simulink model "OMAP_ver_MIL10"  (R2018b)
settings: Solver=FixedStepDiscrete  StartTime=0.0  StopTime=10.0  FixedStep=0.01  RelTol=1e-3
undefined symbols (not defined in the file or in its folder): OMAP_Switch_EMS, OMAP_Switch_EPS, OMAP_Switch_ESC, OMAP_Switch_IC, OMAP_Switch_OTHER, TH_HMIClb_tiDgrdIconWarnHiDurT_C, TH_HMIClb_tiDgrdIconWarnLoDurT_C, TH_HMIClb_tiDgrdVocWarnDurT_C, TH_HMIClb_tiHndOffTxtWarnT_C, TH_HMIClb_tiHndOffVocWarnT_C, TH_HMIClb_tiSWALimFlgDetT_C, TH_HMIClb_tiTxtLimT_C
libraries: simulink x118
(part 6 of 9)

== system OMAP_ver_MIL10/OMAP_Module/ICA_Direct_G59/ICA_Define/TH_HMIClb ==
  note: Level: 3
      | Num: THC.06
      | Rev: 00.00.01
      | Ud: 19-03-28
  Bus Creator1 : BusCreator  Inputs=15
  Constant : Constant  Value=0.01  OutDataTypeStr=single
  Data Type Conversion{,1..7} (8 alike) : DataTypeConversion  OutDataTypeStr=single
  Data Type Conversion{10..13} (4 alike) : DataTypeConversion  OutDataTypeStr=uint16
  ISA_TYPE : Subsystem
      mask Display:
      | port_label('input', 1, 'In');
      | port_label('output', 1, 'Out');
      | color('blue');
      | text(0.5,0.5,'0.789','horizontalAlignment','center');
  ISA_Value : Subsystem
      mask Display:
      | port_label('input', 1, 'In');
      | port_label('output', 1, 'Out');
      | color('blue');
      | text(0.5,0.5,'0.789','horizontalAlignment','center');
  LCScene_tmp : Subsystem
      mask Display:
      | port_label('input', 1, 'In');
      | port_label('output', 1, 'Out');
      | color('blue');
      | text(0.5,0.5,'0.789','horizontalAlignment','center');
  Mode_tmp : Subsystem
      mask Display:
      | port_label('input', 1, 'In');
      | port_label('output', 1, 'Out');
      | color('blue');
      | text(0.5,0.5,'0.789','horizontalAlignment','center');
  TH_HMIClb_tiDgrdIconWarnHiDurT_C : Subsystem
      mask Display:
      | port_label('input', 1, 'In');
      | port_label('output', 1, 'Out');
      | color('blue');
      | text(0.5,0.5,'0.789','horizontalAlignment','center');
  TH_HMIClb_tiDgrdIconWarnLoDurT_C : Subsystem
      mask Display:
      | port_label('input', 1, 'In');
      | port_label('output', 1, 'Out');
      | color('blue');
      | text(0.5,0.5,'0.789','horizontalAlignment','center');
  TH_HMIClb_tiDgrdVocWarnDurT_C : Subsystem
      mask Display:
      | port_label('input', 1, 'In');
      | port_label('output', 1, 'Out');
      | color('blue');
      | text(0.5,0.5,'0.789','horizontalAlignment','center');
  "TH_HMIClb_tiHndOffTxtWarnT_C " : Subsystem
      mask Display:
      | port_label('input', 1, 'In');
      | port_label('output', 1, 'Out');
      | color('blue');
      | text(0.5,0.5,'0.789','horizontalAlignment','center');
  TH_HMIClb_tiHndOffVocWarnT_C : Subsystem
      mask Display:
      | port_label('input', 1, 'In');
      | port_label('output', 1, 'Out');
      | color('blue');
      | text(0.5,0.5,'0.789','horizontalAlignment','center');
  TH_HMIClb_tiSWALimFlgDetT_C : Subsystem
      mask Display:
      | port_label('input', 1, 'In');
      | port_label('output', 1, 'Out');
      | color('blue');
      | text(0.5,0.5,'0.789','horizontalAlignment','center');
  TH_HMIClb_tiTxtLimT_C : Subsystem
      mask Display:
      | port_label('input', 1, 'In');
      | port_label('output', 1, 'Out');
      | color('blue');
      | text(0.5,0.5,'0.789','horizontalAlignment','center');
  Out : Outport
  wires:
  Bus Creator1/1 -> Out/1
  "TH_HMIClb_tiHndOffTxtWarnT_C "/1(Out1) -> Bus Creator1/1  "TH_HMIClb_tiHndOffTxtWarnT_C"
  Data Type Conversion3/1 -> "TH_HMIClb_tiHndOffTxtWarnT_C "/1(In2)
  TH_HMIClb_tiHndOffVocWarnT_C/1(Out1) -> Bus Creator1/2  "TH_HMIClb_tiHndOffVocWarnT_C"
  Data Type Conversion1/1 -> TH_HMIClb_tiHndOffVocWarnT_C/1(In2)
  TH_HMIClb_tiDgrdVocWarnDurT_C/1(Out1) -> Bus Creator1/3  "TH_HMIClb_tiDgrdVocWarnDurT_C"
  Data Type Conversion2/1 -> TH_HMIClb_tiDgrdVocWarnDurT_C/1(In2)
  TH_HMIClb_tiTxtLimT_C/1(Out1) -> Bus Creator1/4  "TH_HMIClb_tiTxtLimT_C"
  Data Type Conversion4/1 -> TH_HMIClb_tiTxtLimT_C/1(In2)
  Data Type Conversion/1 -> Bus Creator1/5  "TH_HMIClb_tiCalcPer_C"
  TH_HMIClb_tiDgrdIconWarnHiDurT_C/1(Out1) -> Bus Creator1/6  "TH_HMIClb_tiDgrdIconWarnHiDurT_C"
  Data Type Conversion5/1 -> TH_HMIClb_tiDgrdIconWarnHiDurT_C/1(In2)
  TH_HMIClb_tiDgrdIconWarnLoDurT_C/1(Out1) -> Bus Creator1/7  "TH_HMIClb_tiDgrdIconWarnLoDurT_C"
  Data Type Conversion6/1 -> TH_HMIClb_tiDgrdIconWarnLoDurT_C/1(In2)
  TH_HMIClb_tiSWALimFlgDetT_C/1(Out1) -> Bus Creator1/8  "TH_HMIClb_tiSWALimFlgDetT_C"
  Data Type Conversion7/1 -> TH_HMIClb_tiSWALimFlgDetT_C/1(In2)
  LCScene_tmp/1(Out1) -> Bus Creator1/11  "LCScene_tmp"
  Data Type Conversion10/1 -> LCScene_tmp/1(In2)  "LCScene_tmp"
  Data Type Conversion12/1 -> ISA_TYPE/1(In2)  "ISA_TYPE"
  ISA_TYPE/1(Out1) -> Bus Creator1/13  "ISA_TYPE"
  ISA_Value/1(Out1) -> Bus Creator1/14  "ISA_Value"
  Data Type Conversion13/1 -> ISA_Value/1(In2)  "ISA_Value"
  Mode_tmp/1(Out1) -> Bus Creator1/15  "Mode_tmp"
  Data Type Conversion11/1 -> Mode_tmp/1(In2)
  Constant/1 -> Data Type Conversion/1

== system OMAP_ver_MIL10/OMAP_Module/ACCS_Direct/ACCS_Define/ACC_State_Synthesis(ACC_SS)/If Action Subsystem2 ==
  In1 : Inport
  Action Port : ActionPort  InitializeStates=reset
  Bus Creator : BusCreator  Inputs=15
  Constant : Constant  Value=2.05  OutDataTypeStr=single
  Constant1 : Constant  Value=6.2  OutDataTypeStr=single
  Constant{3,5,7,9..10} (5 alike) : Constant  Value=0  OutDataTypeStr=uint8
  Constant2 : Constant  Value=6.2  OutDataTypeStr=single
  Constant4 : Constant  Value=-4000  OutDataTypeStr=single
  Constant6 : Constant  Value=-4000  OutDataTypeStr=single
  OMAPve_y_ADAS_ACCRequestEPBNum1 : Constant  Value=0  OutDataTypeStr=uint8
  OMAPve_y_ADAS_ESCDriveOffNum : Constant  Value=0  OutDataTypeStr=uint8
  OMAPve_y_ADAS_ESCHoldReq : Constant  Value=0  OutDataTypeStr=uint8
  Signal Conversion : SignalConversion  OverrideOpt=off
  Subsystem : Subsystem
  Subsystem4 : Subsystem
  Control_Ouput : Outport
  wires:
  Signal Conversion/1 -> Control_Ouput/1
  Constant5/1 -> Bus Creator/12  "Power_steering_power_cut3F2"
  Bus Creator/1 -> Signal Conversion/1
  Subsystem/1(Function_Acc_status) -> Bus Creator/6  "Function_Acc_status"
  In1/1 -> Subsystem/1(In1)
  Constant10/1 -> Bus Creator/11  "MDD_deceleration_type"
  Constant9/1 -> Bus Creator/10  "MDD_Decelerationcontrol_request"
  Subsystem4/1(TYPE_RAPPORT) -> Bus Creator/9  "TYPE_RAPPORT"
  Constant7/1 -> Bus Creator/8  "Powertrain_torquewheel_request"
  Constant6/1 -> Bus Creator/7  "ACCTqReq"
  Constant4/1 -> Bus Creator/5  "PotACCTqReq"
  Constant3/1 -> Bus Creator/4  "StAcvTqWhlPTPotReq"
  Constant2/1 -> Bus Creator/3  "TminUpGear"
  Constant1/1 -> Bus Creator/2  "TminDownGear"
  Constant/1 -> Bus Creator/1  "Deceleration_setpoint_device"
  OMAPve_y_ADAS_ESCDriveOffNum/1 -> Bus Creator/13  "OMAPve_y_ADAS_ESCDriveOff"
  OMAPve_y_ADAS_ESCHoldReq/1 -> Bus Creator/14  "OMAPve_y_ADAS_ESCHoldReq"
  OMAPve_y_ADAS_ACCRequestEPBNum1/1 -> Bus Creator/15  "OMAPve_y_ADAS_ACCRequestEPB"

== system OMAP_ver_MIL10/OMAP_Module/ACCS_Direct/ACCS_Define/ACC_State_Synthesis(ACC_SS)/If Action Subsystem3 ==
  ACT_Control_Signal : Inport
  Action Port : ActionPort  InitializeStates=reset
  Bus Creator : BusCreator  Inputs=15
  Bus Selector1 : BusSelector  OutputSignals=ACCSve_g_ACC_TqReq_convert,ACCSve_d_ACC_TqFlag_convert,ACCSve_g_ACC_DecReq_convert,ACCSve_d_ACC_DecFlag_convert,ACCSve_d_ACC_State_convert,ACCSve_d_ACC_ESCDriveOff_convert,ACCSve_d_ACC_ESCHoldReq_convert,ACCSve_d_ACC_EPBReq_convert
  Constant5 : Constant  Value=0  OutDataTypeStr=uint8
  Data Type Conversion{,1..6} (7 alike) : DataTypeConversion  OutDataTypeStr=uint8
  Gain : Gain  OutDataTypeStr=single
  Signal Conversion : SignalConversion  OverrideOpt=off
  Subsystem : Subsystem
  Subsystem1 : Subsystem
  Subsystem2 : Subsystem
  Subsystem3 : Subsystem
  Subsystem5 : Subsystem
  Subsystem6 : Subsystem
  Control_Ouput : Outport
  wires:
  Bus Selector1/4 -> [ESC_Enable]  "<ACCSve_d_ACC_DecFlag_convert>"
  Bus Selector1/3 -> [ESC_DecTar]  "<ACCSve_g_ACC_DecReq_convert>"
  Bus Selector1/2 -> [EMS_Enable]  "<ACCSve_d_ACC_TqFlag_convert>"
  Bus Selector1/1 -> [EMS_DecTar]  "<ACCSve_g_ACC_TqReq_convert>"
  Data Type Conversion2/1 -> Bus Creator/11  "MDD_deceleration_type"
  Data Type Conversion1/1 -> Bus Creator/10  "MDD_Decelerationcontrol_request"
  Data Type Conversion/1 -> Bus Creator/8  "Powertrain_torquewheel_request"
  Subsystem6/1(TYPE_RAPPORT) -> Bus Creator/9  "TYPE_RAPPORT"
  [EMS_Enable] -> Data Type Conversion/1
  Signal Conversion/1 -> Control_Ouput/1
  Constant5/1 -> Bus Creator/12  "Power_steering_power_cut3F2"
  Gain/1 -> Bus Creator/5  "PotACCTqReq"
  [EMS_Enable] -> Subsystem5/2(In2)
  [EMS_DecTar] -> Subsystem5/1(In1)
  Subsystem3/1(Function_Acc_status) -> Bus Creator/6  "Function_Acc_status"
  Bus Selector1/5 -> Data Type Conversion3/1  "<ACCSve_d_ACC_State_convert>"
  Subsystem2/1(StAcvTqWhlPTPotReq) -> Bus Creator/4  "StAcvTqWhlPTPotReq"
  [ESC_Enable] -> Subsystem2/2(In2)
  Subsystem1/1(TminUpGear) -> Bus Creator/3  "TminUpGear"
  Subsystem/1(TminDownGear) -> Bus Creator/2  "TminDownGear"
  [EMS_Enable] -> Subsystem1/1(In1), Subsystem/1(In1), Subsystem2/1(In1)
  ACT_Control_Signal/1 -> Bus Selector1/1
  Bus Creator/1 -> Signal Conversion/1
  [ESC_DecTar] -> Bus Creator/1  "Deceleration_setpoint_device"
  [EMS_DecTar] -> Gain/1, Bus Creator/7  "ACCTqReq"
  [ESC_Enable] -> Data Type Conversion1/1
  [ESC_Enable] -> Data Type Conversion2/1
  Data Type Conversion3/1 -> Subsystem3/1(In1)
  [ESC_Hold] -> Data Type Conversion5/1
  [ESC_EPB] -> Data Type Conversion6/1
  [ESC_DriveOff] -> Data Type Conversion4/1
  Bus Selector1/6 -> [ESC_DriveOff]  "<ACCSve_d_ACC_ESCDriveOff_convert>"
  Bus Selector1/7 -> [ESC_Hold]  "<ACCSve_d_ACC_ESCHoldReq_convert>"
  Bus Selector1/8 -> [ESC_EPB]  "<ACCSve_d_ACC_EPBReq_convert>"
  Data Type Conversion4/1 -> Bus Creator/13  "OMAPve_y_ADAS_ESCDriveOff"
  Data Type Conversion5/1 -> Bus Creator/14  "OMAPve_y_ADAS_ESCHoldReq"
  Data Type Conversion6/1 -> Bus Creator/15  "OMAPve_y_ADAS_ACCRequestEPB"

== system OMAP_ver_MIL10/OMAP_Module/ACCS_Direct/ACCS_Define/Human_Machine_Interface(ACC_HMI)/Subsystem ==
  Distance : Inport
  CIPV_ID : Inport  Port=2
  ACC_State : Inport  Port=3
  Chart : Stateflow chart  TreatAsAtomicUnit=on
  Compare To Constant13 : simulink/Logic and Bit Operations/Compare To Constant  relop=>  const=0  OutDataTypeStr=boolean
  Compare To Constant14 : simulink/Logic and Bit Operations/Compare To Constant  relop===  const=4  OutDataTypeStr=boolean
  Compare To Constant16 : simulink/Logic and Bit Operations/Compare To Constant  relop===  const=7  OutDataTypeStr=boolean
  Compare To Constant17 : simulink/Logic and Bit Operations/Compare To Constant  relop===  const=8  OutDataTypeStr=boolean
  Compare To Constant18 : simulink/Logic and Bit Operations/Compare To Constant  relop===  const=5  OutDataTypeStr=boolean
  Constant : Constant  Value=5  OutDataTypeStr=uint8
  Constant1 : Constant  Value=0  OutDataTypeStr=uint8
  Logical Operator5 : Logic  Operator=OR  Inputs=4  AllPortsSameDT=off  OutDataTypeStr=boolean
  Switch : Switch  Criteria=u2 ~= 0
  Switch1 : Switch  Criteria=u2 ~= 0
  TARGET_POSITION : Outport
  TgDisp_Flag : Outport  Port=2
  wires:
  Distance/1 -> Chart/1(Distance)
  Chart/1(Value) -> Switch/1
  ACC_State/1 -> Compare To Constant16/1, Compare To Constant17/1, Compare To Constant14/1, Compare To Constant18/1
  Compare To Constant18/1 -> Logical Operator5/1
  Compare To Constant14/1 -> Logical Operator5/2
  Compare To Constant16/1 -> Logical Operator5/3
  Compare To Constant17/1 -> Logical Operator5/4
  Logical Operator5/1 -> Switch/2, Switch1/2
  Switch/1 -> TARGET_POSITION/1
  Constant/1 -> Switch/3
  Switch1/1 -> TgDisp_Flag/1
  CIPV_ID/1 -> Compare To Constant13/1
  Compare To Constant13/1 -> Switch1/1
  Constant1/1 -> Switch1/3

== system OMAP_ver_MIL10/OMAP_Module/ACCS_Direct/ACCS_Define/Human_Machine_Interface(ACC_HMI)/Subsystem9 ==
  ACC_State : Inport
  ACCICA_Flag : Inport  Port=2
  VelocitySet : Inport  Port=3
  Bus Creator : BusCreator  Inputs=4
  Bus Selector : BusSelector  OutputSignals=ACC_Vehicle_Icon_Display,ACC_Set_Speed_Display,ACC_DesiredHeadway_Icon_Basic,RVVACC_Vehiclespeed_request_type
  Constant : Constant  Value=0  OutDataTypeStr=uint16
  Multiport Switch : MultiPortSwitch  DataPortOrder=Specify indices  DataPortIndices={0,1,2,3,4,5,6,7,8,15}  DiagnosticForDefault=Warning
  Subsystem : Subsystem
  Subsystem1 : Subsystem
  Subsystem2 : Subsystem
  Subsystem3 : Subsystem
  Subsystem4 : Subsystem
  Subsystem5 : Subsystem
  Subsystem6 : Subsystem
  Subsystem7 : Subsystem
  Subsystem8 : Subsystem
  Switch : Switch  Criteria=u2 ~= 0
  Out1 : Outport
  wires:
  Subsystem/1(Out1) -> Multiport Switch/2, Multiport Switch/3
  Multiport Switch/1 -> Bus Selector/1
  ACC_State/1 -> Multiport Switch/1
  Subsystem2/1(Out1) -> Multiport Switch/5
  Subsystem1/1(Out1) -> Multiport Switch/4
  Subsystem3/1(Out1) -> Multiport Switch/6
  Subsystem4/1(Out1) -> Multiport Switch/7
  Subsystem5/1(Out1) -> Multiport Switch/8
  Subsystem6/1(Out1) -> Multiport Switch/9
  Subsystem7/1(Out1) -> Multiport Switch/10
  Subsystem8/1(Out1) -> Multiport Switch/11
  VelocitySet/1 -> Subsystem2/1(VelocitySet), Subsystem1/1(VelocitySet)
  ACCICA_Flag/1 -> Switch/2
  Constant/1 -> Switch/1
  Bus Creator/1 -> Out1/1
  Bus Selector/1 -> Switch/3  "<ACC_Vehicle_Icon_Display>"
  Bus Selector/2 -> Bus Creator/2  "<ACC_Set_Speed_Display>"
  Bus Selector/3 -> Bus Creator/3  "<ACC_DesiredHeadway_Icon_Basic>"
  Bus Selector/4 -> Bus Creator/4  "<RVVACC_Vehiclespeed_request_type>"
  Switch/1 -> Bus Creator/1  "ACC_Vehicle_Icon_Display"

== system OMAP_ver_MIL10/OMAP_Module/ACCS_Direct/ACCS_Define/Human_Machine_Interface(ACC_HMI)/Text_PopUp ==
  ACC_State : Inport
  ACCICA_Flag : Inport  Port=2
  ACCActive_Signal : Inport  Port=3
  go_request : Inport  Port=4
  ACC_DecReq : Inport  Port=5
  " Radar_Blocked" : Subsystem
  ACC_Activation_Unsatisfied : Subsystem
  ACC_Active : Subsystem
  ACC_Canceled : Subsystem
  ACC_Fault : Subsystem
  ACC_OFF : Subsystem
  ACC_ON : Subsystem
  ACC_go_request : Subsystem
  Cast : DataTypeConversion  OutDataTypeStr=uint8
  Constant : Constant  Value=0  OutDataTypeStr=uint16
  Constant1 : Constant  Value=0  OutDataTypeStr=uint16
  Gain : Gain
  Gain1 : Gain  Gain=10
  Gain2 : Gain  Gain=3
  Gain3 : Gain  Gain=8
  Gain4 : Gain  Gain=5
  Gain5 : Gain  Gain=2
  Gain6 : Gain  Gain=4
  Gain7 : Gain  Gain=7
  Gain9 : Gain  Gain=9
  Please_Take_Over_the_Car : Subsystem
  Please_Take_Over_the_Car_immediataly : Subsystem
  Radar_State : Constant  Value=2
  Switch{1..10} (10 alike) : Switch  Criteria=u2 > Threshold
  Switch11 : Switch  Criteria=u2 ~= 0
  Unit Delay1 : UnitDelay  SampleTime=-1
  gorequest : Gain  Gain=6
  For4F7 : Outport
  ForTJA : Outport  Port=2
  wires:
  ACC_ON/1(Out1) -> Gain/1
  Cast/1 -> " Radar_Blocked"/1(In1)
  " Radar_Blocked"/1(Out1) -> Gain5/1
  ACC_Fault/1(Out1) -> Gain2/1
  ACCActive_Signal/1 -> ACC_Activation_Unsatisfied/2(In2)
  ACC_Activation_Unsatisfied/1(Out1) -> Gain6/1
  ACC_Active/1(Out1) -> Gain4/1
  go_request/1 -> ACC_go_request/1(In1)
  ACC_go_request/1(<GoRequest>) -> gorequest/1
  Please_Take_Over_the_Car/1(Out1) -> Gain7/1
  ACC_State/1 -> ACC_OFF/1(In1), ACC_Canceled/1(In1), Please_Take_Over_the_Car/1(In1), ACC_Active/1(In1), ACC_Activation_Unsatisfied/1(In1), ACC_Fault/1(In1), ACC_ON/1(In1)
  Please_Take_Over_the_Car_immediataly/1(Out1) -> Gain3/1
  ACC_Canceled/1(Out1) -> Gain9/1
  ACC_OFF/1(Out1) -> Gain1/1
  Gain/1 -> Switch1/1, Switch1/2
  Gain5/1 -> Switch2/1, Switch2/2
  Gain2/1 -> Switch3/1, Switch3/2
  Gain6/1 -> Switch4/1, Switch4/2
  Gain4/1 -> Switch5/1, Switch5/2
  gorequest/1 -> Switch6/1, Switch6/2
  Gain7/1 -> Switch7/1, Switch7/2
  Gain3/1 -> Switch8/1, Switch8/2
  Gain9/1 -> Switch9/1, Switch9/2
  Constant/1 -> Switch1/3
  Switch1/1 -> Switch2/3
  Switch2/1 -> Switch3/3
  Switch3/1 -> Switch4/3
  Switch4/1 -> Switch5/3
  Switch5/1 -> Switch6/3
  Switch6/1 -> Switch7/3
  Switch7/1 -> Switch8/3
  Switch8/1 -> Switch9/3
  Gain1/1 -> Switch10/1, Switch10/2
  Switch9/1 -> Switch10/3
  Switch10/1 -> Unit Delay1/1, ForTJA/1, Switch11/3
  [ACCICA_Flag] -> Switch11/2
  Constant1/1 -> Switch11/1
  Switch11/1 -> For4F7/1
  [Text] -> ACC_ON/2(In2)
  Unit Delay1/1 -> [Text]
  [ACCICA_Flag] -> ACC_OFF/2(In2)
  ACCICA_Flag/1 -> [ACCICA_Flag]
  [ACCICA_Flag] -> ACC_ON/3(ACCICA_Flag)
  Radar_State/1 -> Cast/1
  ACC_DecReq/1 -> Please_Take_Over_the_Car_immediataly/1(ESC_DecTar)

== system OMAP_ver_MIL10/OMAP_Module/ICA_Direct_G59/ICA_Define/ICA_EPS/EPS_Ctr_Disable ==
  stEPSCtlState : Inport
  Action Port : ActionPort  InitializeStates=reset
  Constant : Constant  Value=0  OutDataTypeStr=single
  Constant1 : Constant  OutDataTypeStr=uint16
  MATLAB Function : MATLAB Function  TreatAsAtomicUnit=on
  stEPSCtlCMD : Outport
  LKA_TRQ_FACT_REQ : Outport  Port=2
  LKA_OR_LPA_REQ : Outport  Port=3
  wires:
  MATLAB Function/1(stEPSCtlCMD) -> stEPSCtlCMD/1
  stEPSCtlState/1 -> MATLAB Function/1(stEPSCtlState)
  Constant/1 -> LKA_TRQ_FACT_REQ/1  "LKA_TRQ_FACT_REQ"
  Constant1/1 -> LKA_OR_LPA_REQ/1  "LKA_OR_LPA_REQ"

== system OMAP_ver_MIL10/OMAP_Module/ICA_Direct_G59/ICA_Define/ICA_EPS/EPS_Ctr_Enable ==
  stEPSCtlState : Inport
  Action Port : ActionPort  InitializeStates=reset
  Constant : Constant  OutDataTypeStr=single
  Constant1 : Constant  OutDataTypeStr=uint16
  MATLAB Function : MATLAB Function  TreatAsAtomicUnit=on
  stEPSCtlCMD : Outport
  LKA_TRQ_FACT_REQ : Outport  Port=2
  LKA_OR_LPA_REQ : Outport  Port=3
  wires:
  stEPSCtlState/1 -> MATLAB Function/1(stEPSCtlState)
  MATLAB Function/1(stEPSCtlCMD) -> stEPSCtlCMD/1
  Constant/1 -> LKA_TRQ_FACT_REQ/1  "LKA_TRQ_FACT_REQ"
  Constant1/1 -> LKA_OR_LPA_REQ/1  "LKA_OR_LPA_REQ"

== system OMAP_ver_MIL10/OMAP_Module/ICA_Direct_G59/ICA_Define/Subsystem1/Dspl ==
  TxHndOff : Inport
  Dspl_stTkOvStChk : Inport  Port=2
  Dspl_facmL0Ql : Inport  Port=3
  Dspl_facmR0Ql : Inport  Port=4
  Dspl_stVehSty : Inport  Port=5
  Dspl_facmL0Type : Inport  Port=6
  Dspl_facmR0Type : Inport  Port=7
  Dspl_stTHState : Inport  Port=8
  Dspl_bsFromFMCMsg : Inport  Port=9
  Dspl_stTHFKeyState : Inport  Port=10
  DsplPrcs_CIb : Inport  Port=11
  Dspl_tfAddVocCmd : Inport  Port=12
  DsplPrcs_dDgrdIconWarnflag : Inport  Port=13
  DsplPrcs_stSWALimFlg : Inport  Port=14
  Bus Selector5 : BusSelector  OutputSignals=TH_HMIClb_tiHndOffTxtWarnT_C,TH_HMIClb_tiDgrdVocWarnDurT_C,TH_HMIClb_tiHndOffVocWarnT_C,TH_HMIClb_tiTxtLimT_C,TH_HMIClb_tiDgrdIconWarnHiDurT_C,TH_HMIClb_tiDgrdIconWarnLoDurT_C,TH_HMIClb_tiSWALimFlgDetT_C,TH_HMIClb_tiCalcPer_C
  Data Type Conversion{,1..5} (6 alike) : DataTypeConversion  OutDataTypeStr=single
  DsplPrcs : Subsystem
  TimePrcs : Subsystem
  Dspl_stTxtDspl : Outport
  Dspl_stIconDspl : Outport  Port=2
  Dspl_stLaneDspl : Outport  Port=3
  Dspl_stL0DispType : Outport  Port=4
  Dspl_stR0DispType : Outport  Port=5
  Dspl_stVocDspl : Outport  Port=6
  Dspl_bsMon : Outport  Port=7
  wires:
  Dspl_stTHState/1 -> DsplPrcs/7(DsplPrcs_stTHState)
  Dspl_stTHFKeyState/1 -> DsplPrcs/9(DsplPrcs_stTHFKeyState)
  Dspl_bsFromFMCMsg/1 -> DsplPrcs/8(DsplPrcs_bsFromFMCMsg)
  Data Type Conversion/1 -> Dspl_stTxtDspl/1
  Data Type Conversion1/1 -> Dspl_stIconDspl/1
  Data Type Conversion2/1 -> Dspl_stLaneDspl/1
  DsplPrcs/6(DsplPrcs_stVocDspl) -> Data Type Conversion3/1
  DsplPrcs/1(DsplPrcs_stTxtDspl) -> Data Type Conversion/1
  DsplPrcs/2(DsplPrcs_stIconDspl) -> Data Type Conversion1/1
  Data Type Conversion3/1 -> Dspl_stVocDspl/1
  DsplPrcs/7(DsplPrcs_bsMon) -> Dspl_bsMon/1
  DsplPrcs_CIb/1 -> Bus Selector5/1
  TimePrcs/2(TimePrcs_dDgrdVocWarnDurnum) -> DsplPrcs/14(DsplPrcs_dDgrdVocWarnDurnum)
  TimePrcs/3(TimePrcs_dHndOffVocWarnnum) -> DsplPrcs/15(DsplPrcs_dHndOffVocWarnnum)
  TimePrcs/1(TimePrcs_dHndOffTxtWarnnum) -> DsplPrcs/13(DsplPrcs_dHndOffTxtWarnnum)
  TimePrcs/4(TimePrcs_dTxtLimnum) -> DsplPrcs/16(DsplPrcs_dTxtLimnum)
  Bus Selector5/3 -> TimePrcs/3(TimePrcs_tiHndOffVocWarnT_C)  "<TH_HMIClb_tiHndOffVocWarnT_C>"
  Bus Selector5/8 -> TimePrcs/8(TimePrcs_tiCalcPer_C)  "<TH_HMIClb_tiCalcPer_C>"
  Bus Selector5/4 -> TimePrcs/4(TimePrcs_tiTxtLimT_C)  "<TH_HMIClb_tiTxtLimT_C>"
  Bus Selector5/1 -> TimePrcs/1(TimePrcs_tiHndOffTxtWarnT_C)  "<TH_HMIClb_tiHndOffTxtWarnT_C>"
  Bus Selector5/2 -> TimePrcs/2(TimePrcs_tiDgrdVocWarnDurT_C)  "<TH_HMIClb_tiDgrdVocWarnDurT_C>"
  TxHndOff/1 -> DsplPrcs/1(DsplPrcs_stStWhlHld)
  Dspl_facmL0Ql/1 -> DsplPrcs/3(DsplPrcs_facmL0Ql)
  Dspl_facmR0Ql/1 -> DsplPrcs/4(DsplPrcs_facmR0Ql)
  Dspl_stVehSty/1 -> DsplPrcs/10(DsplPrcs_stVehSty)
  Dspl_tfAddVocCmd/1 -> DsplPrcs/11(DsplPrcs_tfAddVocCmd)
  TimePrcs/5(TimePrcs_dDgrdIconWarnHiDurnum) -> DsplPrcs/17(DsplPrcs_dDgrdIconWarnHiDurnum)
  TimePrcs/6(TimePrcs_dDgrdIconWarnLoDurnum) -> DsplPrcs/18(DsplPrcs_dDgrdIconWarnLoDurnum)
  Bus Selector5/5 -> TimePrcs/5(TimePrcs_tiDgrdIconWarnHiDurT_C)  "<TH_HMIClb_tiDgrdIconWarnHiDurT_C>"
  Bus Selector5/6 -> TimePrcs/6(TimePrcs_tiDgrdIconWarnLoDurT_C)  "<TH_HMIClb_tiDgrdIconWarnLoDurT_C>"
  DsplPrcs_dDgrdIconWarnflag/1 -> DsplPrcs/20(DsplPrcs_dDgrdIconWarnflag)
  DsplPrcs_stSWALimFlg/1 -> DsplPrcs/12(DsplPrcs_stSWALimFlg)
  Bus Selector5/7 -> TimePrcs/7(TimePrcs_tiSWALimFlgDetT_C)  "<TH_HMIClb_tiSWALimFlgDetT_C>"
  TimePrcs/7(TimePrcs_tiSWALimFlgDetnum) -> DsplPrcs/19(DsplPrcs_tiSWALimFlgDetnum)
  Dspl_stTkOvStChk/1 -> DsplPrcs/2(DsplPrcs_stTkOvStChk)
  Dspl_facmL0Type/1 -> DsplPrcs/5(DsplPrcs_facmL0Type)
  Dspl_facmR0Type/1 -> DsplPrcs/6(DsplPrcs_facmR0Type)
  Data Type Conversion4/1 -> Dspl_stL0DispType/1
  Data Type Conversion5/1 -> Dspl_stR0DispType/1
  DsplPrcs/3(DsplPrcs_stLaneDspl) -> Data Type Conversion2/1
  DsplPrcs/4(DsplPrcs_stL0DispType) -> Data Type Conversion4/1
  DsplPrcs/5(DsplPrcs_stR0DispType) -> Data Type Conversion5/1

== system OMAP_ver_MIL10/OMAP_Module/ICA_Direct_G59/ICA_Define/Subsystem1/Subsystem ==
  THMode : Inport
  LCRMode : Inport  Port=2
  Vehicle_Line_Display_Org : Inport  Port=3
  High_Time : Inport  Port=4
  Low_Time : Inport  Port=5
  ISA_Value : Inport  Port=6
  ISA_Type : Inport  Port=7
  LC_Scene : Inport  Port=8
  Compare To Constant : simulink/Logic and Bit Operations/Compare To Constant  relop===  const=uint16(4)  OutDataTypeStr=boolean
  Compare To Constant1 : simulink/Logic and Bit Operations/Compare To Constant  relop===  const=uint16(2)  OutDataTypeStr=boolean
  Compare To Constant2 : simulink/Logic and Bit Operations/Compare To Constant  relop===  const=uint16(3)  OutDataTypeStr=boolean
  Constant4 : Constant  Value=0  OutDataTypeStr=uint16
  Constant5 : Constant  Value=0  OutDataTypeStr=uint16
  Constant6 : Constant  Value=0  OutDataTypeStr=uint16
  Data Type Conversion : DataTypeConversion  OutDataTypeStr=uint16
  Data Type Conversion1 : DataTypeConversion  OutDataTypeStr=uint16
  Gain : Gain  Gain=100
  Gain1 : Gain  Gain=100
  Logical Operator1 : Logic  Operator=OR  AllPortsSameDT=off  OutDataTypeStr=boolean
  MATLAB Function : MATLAB Function  TreatAsAtomicUnit=on
  Subsystem : Subsystem
  Switch{1..3,6} (4 alike) : Switch  Criteria=u2 > Threshold
  TSR_Version_Only_Sign_Type : Outport
  Vehicle_Line_Display : Outport  Port=2
  ISA Value : Outport  Port=3
  wires:
  Vehicle_Line_Display_Org/1 -> Vehicle_Line_Display/1
  Compare To Constant/1 -> Switch1/2
  MATLAB Function/1(TSR_Version_Only_Sign_Type) -> Switch2/1, Switch1/1
  Switch1/1 -> TSR_Version_Only_Sign_Type/1
  Subsystem/1(Signal) -> Switch2/2
  Constant5/1 -> Switch2/3
  Switch2/1 -> Switch3/1
  Constant6/1 -> Switch3/3
  Switch3/1 -> Switch1/3
  Logical Operator1/1 -> Switch3/2
  High_Time/1 -> Gain/1
  Low_Time/1 -> Gain1/1
  Gain/1 -> Data Type Conversion/1
  Gain1/1 -> Data Type Conversion1/1
  Data Type Conversion/1 -> Subsystem/1(HiDurnum)
  Data Type Conversion1/1 -> Subsystem/2(LoDurnum)
  THMode/1 -> [THMode], Compare To Constant/1
  ISA_Value/1 -> Switch6/1, Switch6/2
  Constant4/1 -> Switch6/3
  Switch6/1 -> ISA Value/1
  LC_Scene/1 -> MATLAB Function/2(LC_Scene)
  [THMode] -> MATLAB Function/1(TH_Mode)
  LCRMode/1 -> [stLCRMode], Compare To Constant1/1, Compare To Constant2/1
  Compare To Constant1/1 -> Logical Operator1/1
  Compare To Constant2/1 -> Logical Operator1/2
  [stLCRMode] -> MATLAB Function/3(stLCRMode)

== system OMAP_ver_MIL10/OMAP_Module/ICA_Direct_G59/ICA_Define/TH_HMIClb/ISA_TYPE ==
  In2 : Inport
  Switch : Switch  Criteria=u2 ~= 0  OutDataTypeStr=single
  tmp : Constant  Value=0  OutDataTypeStr=uint16
  Out1 : Outport
  wires:
  In2/1 -> Switch/2, Switch/1
  Switch/1 -> Out1/1
  tmp/1 -> Switch/3

== system OMAP_ver_MIL10/OMAP_Module/ICA_Direct_G59/ICA_Define/TH_HMIClb/ISA_Value ==
  In2 : Inport
  Switch : Switch  Criteria=u2 ~= 0  OutDataTypeStr=single
  tmp : Constant  Value=0  OutDataTypeStr=uint16
  Out1 : Outport
  wires:
  tmp/1 -> Switch/3
  Switch/1 -> Out1/1
  In2/1 -> Switch/1, Switch/2

== system OMAP_ver_MIL10/OMAP_Module/ICA_Direct_G59/ICA_Define/TH_HMIClb/LCScene_tmp ==
  In2 : Inport
  Switch : Switch  Criteria=u2 ~= 0  OutDataTypeStr=single
  tmp : Constant  Value=0  OutDataTypeStr=uint16
  Out1 : Outport
  wires:
  In2/1 -> Switch/2, Switch/1
  Switch/1 -> Out1/1
  tmp/1 -> Switch/3

== system OMAP_ver_MIL10/OMAP_Module/ICA_Direct_G59/ICA_Define/TH_HMIClb/Mode_tmp ==
  In2 : Inport
  Switch : Switch  Criteria=u2 ~= 0  OutDataTypeStr=single
  tmp : Constant  Value=0  OutDataTypeStr=uint16
  Out1 : Outport
  wires:
  tmp/1 -> Switch/3
  Switch/1 -> Out1/1
  In2/1 -> Switch/1, Switch/2

== system OMAP_ver_MIL10/OMAP_Module/ICA_Direct_G59/ICA_Define/TH_HMIClb/TH_HMIClb_tiDgrdIconWarnHiDurT_C ==
  In2 : Inport
  Constant : Constant  Value=TH_HMIClb_tiDgrdIconWarnHiDurT_C  OutDataTypeStr=single
  Switch : Switch  Criteria=u2 ~= 0  OutDataTypeStr=single
  Out1 : Outport
  wires:
  Constant/1 -> Switch/3
  Switch/1 -> Out1/1
  In2/1 -> Switch/1, Switch/2

== system OMAP_ver_MIL10/OMAP_Module/ICA_Direct_G59/ICA_Define/TH_HMIClb/TH_HMIClb_tiDgrdIconWarnLoDurT_C ==
  In2 : Inport
  Constant : Constant  Value=TH_HMIClb_tiDgrdIconWarnLoDurT_C  OutDataTypeStr=single
  Switch : Switch  Criteria=u2 ~= 0  OutDataTypeStr=single
  Out1 : Outport
  wires:
  In2/1 -> Switch/2, Switch/1
  Switch/1 -> Out1/1
  Constant/1 -> Switch/3

== system OMAP_ver_MIL10/OMAP_Module/ICA_Direct_G59/ICA_Define/TH_HMIClb/TH_HMIClb_tiDgrdVocWarnDurT_C ==
  In2 : Inport
  Switch : Switch  Criteria=u2 ~= 0  OutDataTypeStr=single
  TH_MIN_SPEED_UPPER 1 : Constant  Value=TH_HMIClb_tiDgrdVocWarnDurT_C  OutDataTypeStr=single
  Out1 : Outport
  wires:
  In2/1 -> Switch/2, Switch/1
  Switch/1 -> Out1/1
  TH_MIN_SPEED_UPPER 1/1 -> Switch/3

== system OMAP_ver_MIL10/OMAP_Module/ICA_Direct_G59/ICA_Define/TH_HMIClb/TH_HMIClb_tiHndOffTxtWarnT_C  ==
  In2 : Inport
  Switch : Switch  Criteria=u2 ~= 0  OutDataTypeStr=single
  TH_MIN_SPEED_UPPER 1 : Constant  Value=TH_HMIClb_tiHndOffTxtWarnT_C  OutDataTypeStr=single
  Out1 : Outport
  wires:
  In2/1 -> Switch/2, Switch/1
  Switch/1 -> Out1/1
  TH_MIN_SPEED_UPPER 1/1 -> Switch/3

== system OMAP_ver_MIL10/OMAP_Module/ICA_Direct_G59/ICA_Define/TH_HMIClb/TH_HMIClb_tiHndOffVocWarnT_C ==
  In2 : Inport
  Switch : Switch  Criteria=u2 ~= 0  OutDataTypeStr=single
  TH_MIN_SPEED_UPPER 1 : Constant  Value=TH_HMIClb_tiHndOffVocWarnT_C  OutDataTypeStr=single
  Out1 : Outport
  wires:
  TH_MIN_SPEED_UPPER 1/1 -> Switch/3
  Switch/1 -> Out1/1
  In2/1 -> Switch/1, Switch/2

== system OMAP_ver_MIL10/OMAP_Module/ICA_Direct_G59/ICA_Define/TH_HMIClb/TH_HMIClb_tiSWALimFlgDetT_C ==
  In2 : Inport
  Switch : Switch  Criteria=u2 ~= 0  OutDataTypeStr=single
  TH_HMIClb_tiSWALimFlgDetT_C : Constant  Value=TH_HMIClb_tiSWALimFlgDetT_C  OutDataTypeStr=single
  Out1 : Outport
  wires:
  TH_HMIClb_tiSWALimFlgDetT_C/1 -> Switch/3
  Switch/1 -> Out1/1
  In2/1 -> Switch/1, Switch/2

== system OMAP_ver_MIL10/OMAP_Module/ICA_Direct_G59/ICA_Define/TH_HMIClb/TH_HMIClb_tiTxtLimT_C ==
  In2 : Inport
  Constant : Constant  Value=TH_HMIClb_tiTxtLimT_C  OutDataTypeStr=single
  Switch : Switch  Criteria=u2 ~= 0  OutDataTypeStr=single
  Out1 : Outport
  wires:
  In2/1 -> Switch/2, Switch/1
  Switch/1 -> Out1/1
  Constant/1 -> Switch/3

== system OMAP_ver_MIL10/OMAP_Module/ACCS_Direct/ACCS_Define/ACC_State_Synthesis(ACC_SS)/If Action Subsystem2/Subsystem ==
  In1 : Inport
  Add : Sum  Inputs=+++  OutDataTypeStr=uint8
  Compare To Constant1 : simulink/Logic and Bit Operations/Compare To Constant  relop===  const=0  OutDataTypeStr=boolean
  Compare To Constant2 : simulink/Logic and Bit Operations/Compare To Constant  relop===  const=1  OutDataTypeStr=boolean
  Compare To Constant3 : simulink/Logic and Bit Operations/Compare To Constant  relop===  const=15  OutDataTypeStr=boolean
  Compare To Constant5 : simulink/Logic and Bit Operations/Compare To Constant  relop===  const=2  OutDataTypeStr=boolean
  Compare To Constant6 : simulink/Logic and Bit Operations/Compare To Constant  relop===  const=3  OutDataTypeStr=boolean
  Gain : Gain  Gain=3
  Gain1 : Gain  Gain=2
  Gain2 : Gain  Gain=15
  Logical Operator1 : Logic  Operator=OR  Inputs=3  AllPortsSameDT=off  OutDataTypeStr=boolean
  Function_Acc_status : Outport
  wires:
  Gain2/1 -> Add/3
  Compare To Constant3/1 -> Gain2/1
  Add/1 -> Function_Acc_status/1
  Gain/1 -> Add/1
  Compare To Constant1/1 -> Logical Operator1/1
  Compare To Constant5/1 -> Gain1/1
  Gain1/1 -> Add/2
  Compare To Constant6/1 -> Logical Operator1/3
  In1/1 -> Compare To Constant2/1, Compare To Constant1/1, Compare To Constant6/1, Compare To Constant5/1, Compare To Constant3/1
  Logical Operator1/1 -> Gain/1
  Compare To Constant2/1 -> Logical Operator1/2

== system OMAP_ver_MIL10/OMAP_Module/ACCS_Direct/ACCS_Define/ACC_State_Synthesis(ACC_SS)/If Action Subsystem2/Subsystem4 ==
  Chart : Stateflow chart  TreatAsAtomicUnit=on
  TYPE_RAPPORT : Outport
  wires:
  Chart/1(RAPPORT) -> TYPE_RAPPORT/1

== system OMAP_ver_MIL10/OMAP_Module/ACCS_Direct/ACCS_Define/ACC_State_Synthesis(ACC_SS)/If Action Subsystem3/Subsystem ==
  In1 : Inport
  Constant1 : Constant  Value=6.2  OutDataTypeStr=single
  Constant11 : Constant  Value=6.2  OutDataTypeStr=single
  Switch : Switch  Criteria=u2 > Threshold
  TminDownGear : Outport
  wires:
  Switch/1 -> TminDownGear/1
  Constant1/1 -> Switch/1
  Constant11/1 -> Switch/3
  In1/1 -> Switch/2

== system OMAP_ver_MIL10/OMAP_Module/ACCS_Direct/ACCS_Define/ACC_State_Synthesis(ACC_SS)/If Action Subsystem3/Subsystem1 ==
  In1 : Inport
  Constant12 : Constant  Value=6.2  OutDataTypeStr=single
  Constant2 : Constant  Value=6.2  OutDataTypeStr=single
  Switch1 : Switch  Criteria=u2 > Threshold
  TminUpGear : Outport
  wires:
  Switch1/1 -> TminUpGear/1
  In1/1 -> Switch1/2
  Constant2/1 -> Switch1/1
  Constant12/1 -> Switch1/3

== system OMAP_ver_MIL10/OMAP_Module/ACCS_Direct/ACCS_Define/ACC_State_Synthesis(ACC_SS)/If Action Subsystem3/Subsystem2 ==
  In1 : Inport
  In2 : Inport  Port=2
  Constant1 : Constant  Value=2  OutDataTypeStr=uint8
  Constant11 : Constant  OutDataTypeStr=uint8
  Constant2 : Constant  Value=0  OutDataTypeStr=uint8
  Switch : Switch  Criteria=u2 > Threshold
  Switch1 : Switch  Criteria=u2 > Threshold
  StAcvTqWhlPTPotReq : Outport
  wires:
  In1/1 -> Switch1/2
  In2/1 -> Switch/2
  Constant1/1 -> Switch/1
  Constant2/1 -> Switch/3
  Constant11/1 -> Switch1/1
  Switch/1 -> Switch1/3
  Switch1/1 -> StAcvTqWhlPTPotReq/1

== system OMAP_ver_MIL10/OMAP_Module/ACCS_Direct/ACCS_Define/ACC_State_Synthesis(ACC_SS)/If Action Subsystem3/Subsystem3 ==
  In1 : Inport
  Compare To Constant1 : simulink/Logic and Bit Operations/Compare To Constant  relop===  const=8  OutDataTypeStr=boolean
  Compare To Constant2 : simulink/Logic and Bit Operations/Compare To Constant  relop===  const=7  OutDataTypeStr=boolean
  Constant1 : Constant  Value=7  OutDataTypeStr=uint8
  Logical Operator1 : Logic  Operator=OR  AllPortsSameDT=off  OutDataTypeStr=boolean
  Switch : Switch  Criteria=u2 > Threshold
  Function_Acc_status : Outport
  wires:
  Logical Operator1/1 -> Switch/2
  Switch/1 -> Function_Acc_status/1
  In1/1 -> Switch/3, Compare To Constant1/1, Compare To Constant2/1
  Compare To Constant1/1 -> Logical Operator1/2
  Compare To Constant2/1 -> Logical Operator1/1
  Constant1/1 -> Switch/1

== system OMAP_ver_MIL10/OMAP_Module/ACCS_Direct/ACCS_Define/ACC_State_Synthesis(ACC_SS)/If Action Subsystem3/Subsystem5 ==
  In1 : Inport
  In2 : Inport  Port=2
  Constant4 : Constant  Value=-4000  OutDataTypeStr=single
  Switch : Switch  Criteria=u2 > Threshold
  PotACCTqReq : Outport
  wires:
  In2/1 -> Switch/2
  In1/1 -> Switch/1
  Constant4/1 -> Switch/3
  Switch/1 -> PotACCTqReq/1

== system OMAP_ver_MIL10/OMAP_Module/ACCS_Direct/ACCS_Define/ACC_State_Synthesis(ACC_SS)/If Action Subsystem3/Subsystem6 ==
  Chart : Stateflow chart  TreatAsAtomicUnit=on
  TYPE_RAPPORT : Outport
  wires:
  Chart/1(RAPPORT) -> TYPE_RAPPORT/1

== system OMAP_ver_MIL10/OMAP_Module/ACCS_Direct/ACCS_Define/Human_Machine_Interface(ACC_HMI)/Subsystem9/Subsystem ==
  Bus Creator : BusCreator  Inputs=4
  Constant{,1..3} (4 alike) : Constant  Value=0  OutDataTypeStr=uint16
  Out1 : Outport
  wires:
  Constant/1 -> Bus Creator/1  "ACC_Vehicle_Icon_Display"
  Constant1/1 -> Bus Creator/2  "ACC_Set_Speed_Display"
  Bus Creator/1 -> Out1/1
  Constant2/1 -> Bus Creator/4  "RVVACC_Vehiclespeed_request_type"
  Constant3/1 -> Bus Creator/3  "ACC_DesiredHeadway_Icon_Basic"

== system OMAP_ver_MIL10/OMAP_Module/ACCS_Direct/ACCS_Define/Human_Machine_Interface(ACC_HMI)/Subsystem9/Subsystem1 ==
  VelocitySet : Inport
  Bus Creator : BusCreator  Inputs=4
  Compare To Constant : simulink/Logic and Bit Operations/Compare To Constant  relop=>  const=10  OutDataTypeStr=boolean
  Constant : Constant  OutDataTypeStr=uint16
  Constant2 : Constant  Value=0  OutDataTypeStr=uint16
  Constant3 : Constant  OutDataTypeStr=uint16
  Constant4 : Constant  OutDataTypeStr=uint16
  Constant5 : Constant  Value=3  OutDataTypeStr=uint16
  Switch : Switch
  Out1 : Outport
  wires:
  Constant3/1 -> Bus Creator/3  "ACC_DesiredHeadway_Icon_Basic"
  Constant2/1 -> Bus Creator/4  "RVVACC_Vehiclespeed_request_type"
  Bus Creator/1 -> Out1/1
  Switch/1 -> Bus Creator/2  "ACC_Set_Speed_Display"
  Constant/1 -> Bus Creator/1  "ACC_Vehicle_Icon_Display"
  VelocitySet/1 -> Compare To Constant/1
  Compare To Constant/1 -> Switch/2
  Constant4/1 -> Switch/1
  Constant5/1 -> Switch/3

== system OMAP_ver_MIL10/OMAP_Module/ACCS_Direct/ACCS_Define/Human_Machine_Interface(ACC_HMI)/Subsystem9/Subsystem2 ==
  VelocitySet : Inport
  Bus Creator : BusCreator  Inputs=4
  Compare To Constant : simulink/Logic and Bit Operations/Compare To Constant  relop=>  const=10  OutDataTypeStr=boolean
  Constant : Constant  OutDataTypeStr=uint16
  Constant2 : Constant  Value=0  OutDataTypeStr=uint16
  Constant3 : Constant  OutDataTypeStr=uint16
  Constant4 : Constant  Value=2  OutDataTypeStr=uint16
  Constant5 : Constant  Value=3  OutDataTypeStr=uint16
  Switch : Switch
  Out1 : Outport
  wires:
  Constant/1 -> Bus Creator/1  "ACC_Vehicle_Icon_Display"
  Switch/1 -> Bus Creator/2  "ACC_Set_Speed_Display"
  Bus Creator/1 -> Out1/1
  Constant2/1 -> Bus Creator/4  "RVVACC_Vehiclespeed_request_type"
  Constant3/1 -> Bus Creator/3  "ACC_DesiredHeadway_Icon_Basic"
  VelocitySet/1 -> Compare To Constant/1
  Compare To Constant/1 -> Switch/2
  Constant4/1 -> Switch/1
  Constant5/1 -> Switch/3

== system OMAP_ver_MIL10/OMAP_Module/ACCS_Direct/ACCS_Define/Human_Machine_Interface(ACC_HMI)/Subsystem9/Subsystem3 ==
  Bus Creator : BusCreator  Inputs=4
  Constant : Constant  Value=2  OutDataTypeStr=uint16
  Constant1 : Constant  Value=2  OutDataTypeStr=uint16
  Constant2 : Constant  OutDataTypeStr=uint16
  Constant3 : Constant  OutDataTypeStr=uint16
  Out1 : Outport
  wires:
  Constant3/1 -> Bus Creator/3  "ACC_DesiredHeadway_Icon_Basic"
  Constant2/1 -> Bus Creator/4  "RVVACC_Vehiclespeed_request_type"
  Bus Creator/1 -> Out1/1
  Constant1/1 -> Bus Creator/2  "ACC_Set_Speed_Display"
  Constant/1 -> Bus Creator/1  "ACC_Vehicle_Icon_Display"

== system OMAP_ver_MIL10/OMAP_Module/ACCS_Direct/ACCS_Define/Human_Machine_Interface(ACC_HMI)/Subsystem9/Subsystem4 ==
  Bus Creator : BusCreator  Inputs=4
  Constant : Constant  Value=2  OutDataTypeStr=uint16
  Constant1 : Constant  Value=4  OutDataTypeStr=uint16
  Constant2 : Constant  OutDataTypeStr=uint16
  Constant3 : Constant  OutDataTypeStr=uint16
  Out1 : Outport
  wires:
  Constant/1 -> Bus Creator/1  "ACC_Vehicle_Icon_Display"
  Constant1/1 -> Bus Creator/2  "ACC_Set_Speed_Display"
  Bus Creator/1 -> Out1/1
  Constant2/1 -> Bus Creator/4  "RVVACC_Vehiclespeed_request_type"
  Constant3/1 -> Bus Creator/3  "ACC_DesiredHeadway_Icon_Basic"

== system OMAP_ver_MIL10/OMAP_Module/ACCS_Direct/ACCS_Define/Human_Machine_Interface(ACC_HMI)/Subsystem9/Subsystem5 ==
  Bus Creator : BusCreator  Inputs=4
  Constant : Constant  Value=2  OutDataTypeStr=uint16
  Constant1 : Constant  Value=2  OutDataTypeStr=uint16
  Constant2 : Constant  OutDataTypeStr=uint16
  Constant3 : Constant  OutDataTypeStr=uint16
  Out1 : Outport
  wires:
  Constant3/1 -> Bus Creator/3  "ACC_DesiredHeadway_Icon_Basic"
  Constant2/1 -> Bus Creator/4  "RVVACC_Vehiclespeed_request_type"
  Bus Creator/1 -> Out1/1
  Constant1/1 -> Bus Creator/2  "ACC_Set_Speed_Display"
  Constant/1 -> Bus Creator/1  "ACC_Vehicle_Icon_Display"

== system OMAP_ver_MIL10/OMAP_Module/ACCS_Direct/ACCS_Define/Human_Machine_Interface(ACC_HMI)/Subsystem9/Subsystem6 ==
  Bus Creator : BusCreator  Inputs=4
  Constant : Constant  Value=2  OutDataTypeStr=uint16
  Constant1 : Constant  Value=2  OutDataTypeStr=uint16
  Constant2 : Constant  Value=0  OutDataTypeStr=uint16
  Constant3 : Constant  OutDataTypeStr=uint16
  Out1 : Outport
  wires:
  Constant/1 -> Bus Creator/1  "ACC_Vehicle_Icon_Display"
  Constant1/1 -> Bus Creator/2  "ACC_Set_Speed_Display"
  Bus Creator/1 -> Out1/1
  Constant2/1 -> Bus Creator/4  "RVVACC_Vehiclespeed_request_type"
  Constant3/1 -> Bus Creator/3  "ACC_DesiredHeadway_Icon_Basic"

== system OMAP_ver_MIL10/OMAP_Module/ACCS_Direct/ACCS_Define/Human_Machine_Interface(ACC_HMI)/Subsystem9/Subsystem7 ==
  Bus Creator : BusCreator  Inputs=4
  Constant : Constant  Value=2  OutDataTypeStr=uint16
  Constant1 : Constant  Value=2  OutDataTypeStr=uint16
  Constant2 : Constant  Value=0  OutDataTypeStr=uint16
  Constant3 : Constant  OutDataTypeStr=uint16
  Out1 : Outport
  wires:
  Constant3/1 -> Bus Creator/3  "ACC_DesiredHeadway_Icon_Basic"
  Constant2/1 -> Bus Creator/4  "RVVACC_Vehiclespeed_request_type"
  Bus Creator/1 -> Out1/1
  Constant1/1 -> Bus Creator/2  "ACC_Set_Speed_Display"
  Constant/1 -> Bus Creator/1  "ACC_Vehicle_Icon_Display"

== system OMAP_ver_MIL10/OMAP_Module/ACCS_Direct/ACCS_Define/Human_Machine_Interface(ACC_HMI)/Subsystem9/Subsystem8 ==
  Bus Creator : BusCreator  Inputs=4
  Constant : Constant  Value=3  OutDataTypeStr=uint16
  Constant1 : Constant  Value=3  OutDataTypeStr=uint16
  Constant2 : Constant  Value=0  OutDataTypeStr=uint16
  Constant3 : Constant  Value=0  OutDataTypeStr=uint16
  Out1 : Outport
  wires:
  Constant/1 -> Bus Creator/1  "ACC_Vehicle_Icon_Display"
  Constant1/1 -> Bus Creator/2  "ACC_Set_Speed_Display"
  Bus Creator/1 -> Out1/1
  Constant2/1 -> Bus Creator/4  "RVVACC_Vehiclespeed_request_type"
  Constant3/1 -> Bus Creator/3  "ACC_DesiredHeadway_Icon_Basic"

== system OMAP_ver_MIL10/OMAP_Module/ACCS_Direct/ACCS_Define/Human_Machine_Interface(ACC_HMI)/Text_PopUp/ Radar_Blocked ==
  In1 : Inport
  Chart : Stateflow chart  TreatAsAtomicUnit=on
  Compare To Constant1 : simulink/Logic and Bit Operations/Compare To Constant  relop=~=  const=6  OutDataTypeStr=boolean
  Compare To Constant15 : simulink/Logic and Bit Operations/Compare To Constant  relop===  const=6  OutDataTypeStr=boolean
  Logical Operator : Logic  AllPortsSameDT=off  OutDataTypeStr=boolean
  Unit Delay : UnitDelay  SampleTime=-1
  Out1 : Outport
  wires:
  In1/1 -> Compare To Constant15/1, Unit Delay/1
  Compare To Constant15/1 -> Logical Operator/2
  Unit Delay/1 -> Compare To Constant1/1
  Compare To Constant1/1 -> Logical Operator/1
  Logical Operator/1 -> Chart/1(data)
  Chart/1(Value) -> Out1/1

== system OMAP_ver_MIL10/OMAP_Module/ACCS_Direct/ACCS_Define/Human_Machine_Interface(ACC_HMI)/Text_PopUp/ACC_Activation_Unsatisfied ==
  In1 : Inport
  In2 : Inport  Port=2
  Chart : Stateflow chart  TreatAsAtomicUnit=on
  Compare To Constant17 : simulink/Logic and Bit Operations/Compare To Constant  relop===  const=2  OutDataTypeStr=boolean
  Logical Operator8 : Logic  AllPortsSameDT=off  OutDataTypeStr=boolean
  Out1 : Outport
  wires:
  Compare To Constant17/1 -> Logical Operator8/1
  In2/1 -> Logical Operator8/2
  Logical Operator8/1 -> Chart/1(data)
  In1/1 -> Compare To Constant17/1
  Chart/1(Value) -> Out1/1

== system OMAP_ver_MIL10/OMAP_Module/ACCS_Direct/ACCS_Define/Human_Machine_Interface(ACC_HMI)/Text_PopUp/ACC_Active ==
  In1 : Inport
  Chart : Stateflow chart  TreatAsAtomicUnit=on
  Compare To Constant12 : simulink/Logic and Bit Operations/Compare To Constant  relop===  const=3  OutDataTypeStr=boolean
  Compare To Constant13 : simulink/Logic and Bit Operations/Compare To Constant  relop===  const=4  OutDataTypeStr=boolean
  Logical Operator6 : Logic  AllPortsSameDT=off  OutDataTypeStr=boolean
  Unit Delay1 : UnitDelay  SampleTime=-1
  Out1 : Outport
  wires:
  Unit Delay1/1 -> Compare To Constant12/1
  In1/1 -> Unit Delay1/1, Compare To Constant13/1
  Compare To Constant12/1 -> Logical Operator6/1
  Compare To Constant13/1 -> Logical Operator6/2
  Logical Operator6/1 -> Chart/1(data)
  Chart/1(Value) -> Out1/1

== system OMAP_ver_MIL10/OMAP_Module/ACCS_Direct/ACCS_Define/Human_Machine_Interface(ACC_HMI)/Text_PopUp/ACC_Canceled ==
  In1 : Inport
  Chart : Stateflow chart  TreatAsAtomicUnit=on
  Compare To Constant1 : simulink/Logic and Bit Operations/Compare To Constant  relop===  const=2  OutDataTypeStr=boolean
  Compare To Constant2 : simulink/Logic and Bit Operations/Compare To Constant  relop===  const=3  OutDataTypeStr=boolean
  Compare To Constant23 : simulink/Logic and Bit Operations/Compare To Constant  relop===  const=4  OutDataTypeStr=boolean
  Compare To Constant3 : simulink/Logic and Bit Operations/Compare To Constant  relop===  const=7  OutDataTypeStr=boolean
  Compare To Constant4 : simulink/Logic and Bit Operations/Compare To Constant  relop===  const=6  OutDataTypeStr=boolean
  Compare To Constant5 : simulink/Logic and Bit Operations/Compare To Constant  relop===  const=2  OutDataTypeStr=boolean
  Compare To Constant6 : simulink/Logic and Bit Operations/Compare To Constant  relop===  const=3  OutDataTypeStr=boolean
  Compare To Constant7 : simulink/Logic and Bit Operations/Compare To Constant  relop===  const=5  OutDataTypeStr=boolean
  Logical Operator1 : Logic  Operator=OR  Inputs=3  AllPortsSameDT=off  OutDataTypeStr=boolean
  Logical Operator16 : Logic  AllPortsSameDT=off  OutDataTypeStr=boolean
  Logical Operator2 : Logic  Operator=OR  AllPortsSameDT=off  OutDataTypeStr=boolean
  Logical Operator3 : Logic  Operator=OR  AllPortsSameDT=off  OutDataTypeStr=boolean
  Logical Operator4 : Logic  AllPortsSameDT=off  OutDataTypeStr=boolean
  Logical Operator5 : Logic  Operator=OR  AllPortsSameDT=off  OutDataTypeStr=boolean
  Unit Delay1 : UnitDelay  SampleTime=-1
  Unit Delay5 : UnitDelay  SampleTime=-1
  Out1 : Outport
  wires:
  Compare To Constant1/1 -> Logical Operator1/1
  Compare To Constant23/1 -> Logical Operator16/1
  Logical Operator16/1 -> Logical Operator2/1
  Chart/1(Value) -> Out1/1
  Unit Delay5/1 -> Compare To Constant23/1
  Compare To Constant2/1 -> Logical Operator1/2
  Compare To Constant3/1 -> Logical Operator1/3
  Logical Operator1/1 -> Logical Operator16/2
  Compare To Constant5/1 -> Logical Operator3/1
  Compare To Constant7/1 -> Logical Operator5/1
  In1/1 -> Compare To Constant6/1, Compare To Constant5/1, Unit Delay1/1, Compare To Constant3/1, Compare To Constant2/1, Compare To Constant1/1, Unit Delay5/1
  Unit Delay1/1 -> Compare To Constant4/1, Compare To Constant7/1
  Compare To Constant6/1 -> Logical Operator3/2
  Logical Operator3/1 -> Logical Operator4/2
  Logical Operator4/1 -> Logical Operator2/2
  Logical Operator2/1 -> Chart/1(data)
  Compare To Constant4/1 -> Logical Operator5/2
  Logical Operator5/1 -> Logical Operator4/1

== system OMAP_ver_MIL10/OMAP_Module/ACCS_Direct/ACCS_Define/Human_Machine_Interface(ACC_HMI)/Text_PopUp/ACC_Fault ==
  In1 : Inport
  Chart : Stateflow chart  TreatAsAtomicUnit=on
  Compare To Constant1 : simulink/Logic and Bit Operations/Compare To Constant  relop=~=  const=15  OutDataTypeStr=boolean
  Compare To Constant15 : simulink/Logic and Bit Operations/Compare To Constant  relop===  const=15  OutDataTypeStr=boolean
  Logical Operator : Logic  AllPortsSameDT=off  OutDataTypeStr=boolean
  Unit Delay : UnitDelay  SampleTime=-1
  Out1 : Outport
  wires:
  Logical Operator/1 -> Chart/1(data)
  In1/1 -> Compare To Constant15/1, Unit Delay/1
  Compare To Constant1/1 -> Logical Operator/1
  Compare To Constant15/1 -> Logical Operator/2
  Unit Delay/1 -> Compare To Constant1/1
  Chart/1(Value) -> Out1/1

== system OMAP_ver_MIL10/OMAP_Module/ACCS_Direct/ACCS_Define/Human_Machine_Interface(ACC_HMI)/Text_PopUp/ACC_OFF ==
  In1 : Inport
  In2 : Inport  Port=2
  Chart : Stateflow chart  TreatAsAtomicUnit=on
  Compare To Constant1 : simulink/Logic and Bit Operations/Compare To Constant  relop===  const=1  OutDataTypeStr=boolean
  Compare To Constant10 : simulink/Logic and Bit Operations/Compare To Constant  relop===  const=8  OutDataTypeStr=boolean
  Compare To Constant2 : simulink/Logic and Bit Operations/Compare To Constant  relop=~=  const=0  OutDataTypeStr=boolean
  Compare To Constant3 : simulink/Logic and Bit Operations/Compare To Constant  relop=~=  const=15  OutDataTypeStr=boolean
  Compare To Constant4 : simulink/Logic and Bit Operations/Compare To Constant  relop=~=  const=1  OutDataTypeStr=boolean
  Compare To Constant5 : simulink/Logic and Bit Operations/Compare To Constant  relop=~=  const=8  OutDataTypeStr=boolean
  Compare To Constant6 : simulink/Logic and Bit Operations/Compare To Constant  relop===  const=0  OutDataTypeStr=boolean
  Compare To Constant7 : simulink/Logic and Bit Operations/Compare To Constant  relop===  const=1  OutDataTypeStr=boolean
  Compare To Constant8 : simulink/Logic and Bit Operations/Compare To Constant  relop===  const=4  OutDataTypeStr=boolean
  Logical Operator1 : Logic  Inputs=4  AllPortsSameDT=off  OutDataTypeStr=boolean
  Logical Operator2 : Logic  AllPortsSameDT=off  OutDataTypeStr=boolean
  Logical Operator3 : Logic  AllPortsSameDT=off  OutDataTypeStr=boolean
  Logical Operator4 : Logic  Operator=OR  AllPortsSameDT=off  OutDataTypeStr=boolean
  Logical Operator5 : Logic  AllPortsSameDT=off  OutDataTypeStr=boolean
  Unit Delay1 : UnitDelay  SampleTime=-1
  Unit Delay2 : UnitDelay  SampleTime=-1
  Unit Delay6 : UnitDelay  SampleTime=-1
  Out1 : Outport
  wires:
  Unit Delay6/1 -> Compare To Constant8/1
  Logical Operator3/1 -> Logical Operator4/1
  Compare To Constant10/1 -> Logical Operator3/2
  Compare To Constant8/1 -> Logical Operator3/1
  Chart/1(Value) -> Out1/1
  Unit Delay1/1 -> Compare To Constant5/1, Compare To Constant4/1, Compare To Constant3/1, Compare To Constant2/1
  Compare To Constant1/1 -> Logical Operator2/2
  Compare To Constant2/1 -> Logical Operator1/1
  In1/1 -> Unit Delay1/1, Compare To Constant1/1, Compare To Constant10/1, Unit Delay6/1
  Compare To Constant3/1 -> Logical Operator1/2
  Compare To Constant4/1 -> Logical Operator1/3
  Compare To Constant5/1 -> Logical Operator1/4
  Logical Operator1/1 -> Logical Operator2/1
  Logical Operator2/1 -> Logical Operator4/2
  Logical Operator4/1 -> Chart/1(data)
  In2/1 -> Unit Delay2/1, Compare To Constant6/1
  Compare To Constant7/1 -> Logical Operator5/1
  Compare To Constant6/1 -> Logical Operator5/2
  Unit Delay2/1 -> Compare To Constant7/1
  Logical Operator5/1 -> Chart/2(data1)
